simulink model "kinematic_obstacle_mpc"  (R2015b)
settings: Solver=FixedStepAuto  StartTime=0.0  StopTime=10.0  FixedStep=0.01  RelTol=1e-3
values from neighbouring files (symbols this model uses):
  goalX = 10    [KINEMATIC_MOTION_PLANNER.m]    (also in KINEMATIC_MOTION_PLANNER2.m = 15)
  goalY = 0    [KINEMATIC_MOTION_PLANNER.m]    (also in KINEMATIC_MOTION_PLANNER2.m)
  Lf = 1    [KINEMATIC_MOTION_PLANNER.m]    (also in KINEMATIC_MOTION_PLANNER2.m; KINEMATIC_STEP_MPC.m; KINEMATIC_VEHICLE_CONTROL.m; KINEMATIC_VEHICLE_SIM.m)
  Lr = 1    [KINEMATIC_MOTION_PLANNER.m]    (also in KINEMATIC_MOTION_PLANNER2.m; KINEMATIC_STEP_MPC.m; KINEMATIC_VEHICLE_CONTROL.m; KINEMATIC_VEHICLE_SIM.m)
  ObstacleX = 5    [KINEMATIC_MOTION_PLANNER.m]    (also in KINEMATIC_MOTION_PLANNER2.m = [5, 8,11])
  ObstacleY = 0    [KINEMATIC_MOTION_PLANNER.m]    (also in KINEMATIC_MOTION_PLANNER2.m = [0,-2.5,0])
  Psi0 = 0    [KINEMATIC_MOTION_PLANNER.m]    (also in KINEMATIC_MOTION_PLANNER2.m; KINEMATIC_STEP_MPC.m; KINEMATIC_VEHICLE_CONTROL.m; KINEMATIC_VEHICLE_SIM.m)
  V = 1    [KINEMATIC_MOTION_PLANNER.m]    (also in KINEMATIC_MOTION_PLANNER2.m; KINEMATIC_STEP_MPC.m; KINEMATIC_VEHICLE_CONTROL.m; KINEMATIC_VEHICLE_SIM.m = 5)
  X0 = 0    [KINEMATIC_MOTION_PLANNER.m]    (also in KINEMATIC_MOTION_PLANNER2.m; KINEMATIC_STEP_MPC.m; KINEMATIC_VEHICLE_CONTROL.m; KINEMATIC_VEHICLE_SIM.m)
  Y0 = 0    [KINEMATIC_MOTION_PLANNER.m]    (also in KINEMATIC_MOTION_PLANNER2.m; KINEMATIC_STEP_MPC.m; KINEMATIC_VEHICLE_CONTROL.m; KINEMATIC_VEHICLE_SIM.m)
settings Model: Creator=gebruiker  LastModifiedBy=gebruiker

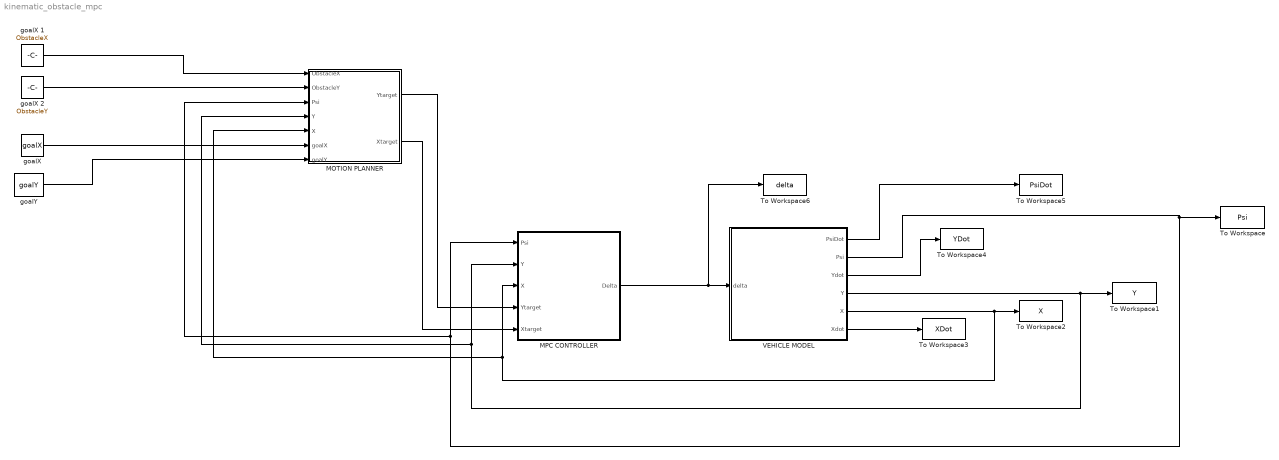
== system kinematic_obstacle_mpc ==
  MOTION PLANNER : Subsystem
  MPC CONTROLLER : Subsystem
  To Workspace : ToWorkspace  VariableName=Psi  SaveFormat=Structure With Time  SampleTime=-1
  To Workspace1 : ToWorkspace  VariableName=Y  SaveFormat=Structure With Time  SampleTime=-1
  To Workspace2 : ToWorkspace  VariableName=X  SaveFormat=Structure With Time  SampleTime=-1
  To Workspace3 : ToWorkspace  VariableName=XDot  SaveFormat=Structure With Time  SampleTime=-1
  To Workspace4 : ToWorkspace  VariableName=YDot  SaveFormat=Structure With Time  SampleTime=-1
  To Workspace5 : ToWorkspace  VariableName=PsiDot  SaveFormat=Structure With Time  SampleTime=-1
  To Workspace6 : ToWorkspace  VariableName=delta  SaveFormat=Structure With Time  SampleTime=-1
  VEHICLE MODEL : Subsystem
  "goalX " : Constant  Value=goalX
  goalX 1 : Constant  Value=ObstacleX
  goalX 2 : Constant  Value=ObstacleY
  "goalY " : Constant  Value=goalY
  wires:
  VEHICLE MODEL/1(PsiDot) -> To Workspace5/1
  VEHICLE MODEL/2(Psi) -> To Workspace/1, MOTION PLANNER/3("Psi "), MPC CONTROLLER/1(Psi)
  VEHICLE MODEL/3(Ydot) -> To Workspace4/1
  VEHICLE MODEL/4(Y) -> MOTION PLANNER/4("Y "), MPC CONTROLLER/2(Y), To Workspace1/1
  VEHICLE MODEL/6(Xdot) -> To Workspace3/1
  MPC CONTROLLER/1(Delta) -> To Workspace6/1, VEHICLE MODEL/1("delta ")
  VEHICLE MODEL/5(X) -> To Workspace2/1, MOTION PLANNER/5(X), MPC CONTROLLER/3(X)
  MOTION PLANNER/1(Ytarget) -> MPC CONTROLLER/4(Ytarget)
  MOTION PLANNER/2(Xtarget) -> MPC CONTROLLER/5(Xtarget)
  "goalX "/1 -> MOTION PLANNER/6(goalX)
  "goalY "/1 -> MOTION PLANNER/7("goalY ")
  goalX 2/1 -> MOTION PLANNER/2(ObstacleY)
  goalX 1/1 -> MOTION PLANNER/1(ObstacleX)

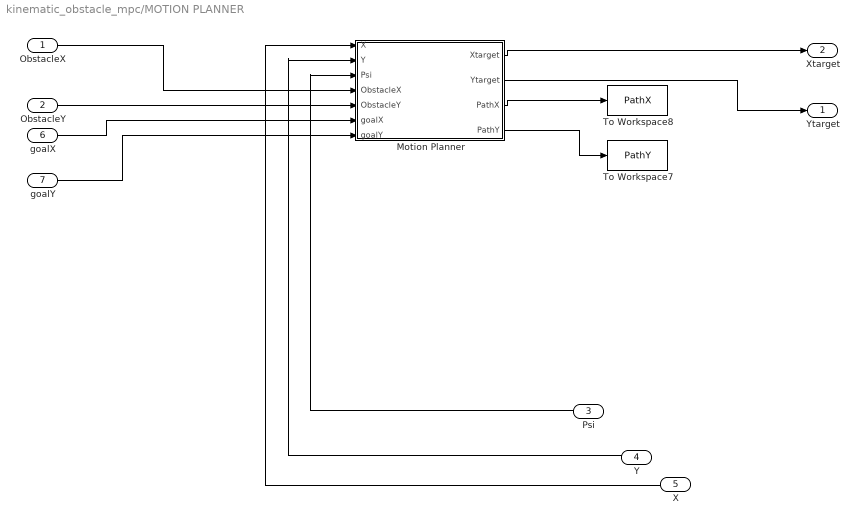
== system kinematic_obstacle_mpc/MOTION PLANNER ==
  ObstacleX : Inport
  ObstacleY : Inport  Port=2
  "Psi " : Inport  Port=3
  "Y " : Inport  Port=4
  X : Inport  Port=5
  goalX : Inport  Port=6
  "goalY " : Inport  Port=7
  Motion Planner : MATLAB Function  TreatAsAtomicUnit=on
  To Workspace7 : ToWorkspace  VariableName=PathY  SaveFormat=Structure With Time  SampleTime=-1
  To Workspace8 : ToWorkspace  VariableName=PathX  SaveFormat=Structure With Time  SampleTime=-1
  Ytarget : Outport
  Xtarget : Outport  Port=2
  wires:
  ObstacleY/1 -> Motion Planner/5(ObstacleY)
  Motion Planner/4(PathY) -> To Workspace7/1
  "Psi "/1 -> Motion Planner/3(Psi)
  "Y "/1 -> Motion Planner/2(Y)
  X/1 -> Motion Planner/1(X)
  Motion Planner/3(PathX) -> To Workspace8/1
  ObstacleX/1 -> Motion Planner/4(ObstacleX)
  Motion Planner/1(Xtarget) -> Xtarget/1
  Motion Planner/2(Ytarget) -> Ytarget/1
  goalX/1 -> Motion Planner/6(goalX)
  "goalY "/1 -> Motion Planner/7(goalY)

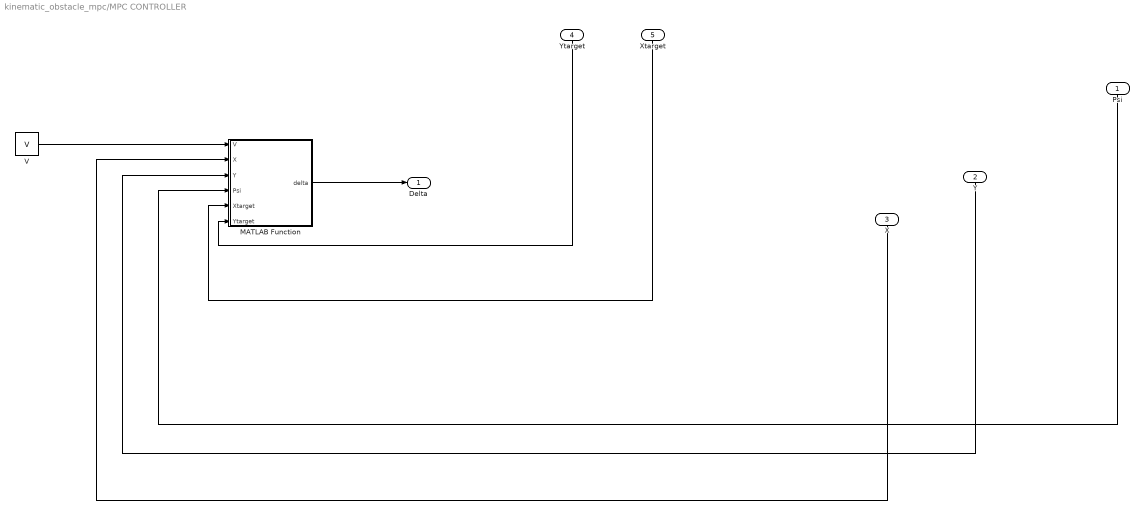
== system kinematic_obstacle_mpc/MPC CONTROLLER ==
  Psi : Inport
  Y : Inport  Port=2
  X : Inport  Port=3
  Ytarget : Inport  Port=4
  Xtarget : Inport  Port=5
  MATLAB Function : MATLAB Function  TreatAsAtomicUnit=on
  "V " : Constant  Value=V
  Delta : Outport
  wires:
  "V "/1 -> MATLAB Function/1(V)
  Y/1 -> MATLAB Function/3(Y)
  Psi/1 -> MATLAB Function/4(Psi)
  X/1 -> MATLAB Function/2(X)
  MATLAB Function/1(delta) -> Delta/1
  Xtarget/1 -> MATLAB Function/5(Xtarget)
  Ytarget/1 -> MATLAB Function/6(Ytarget)

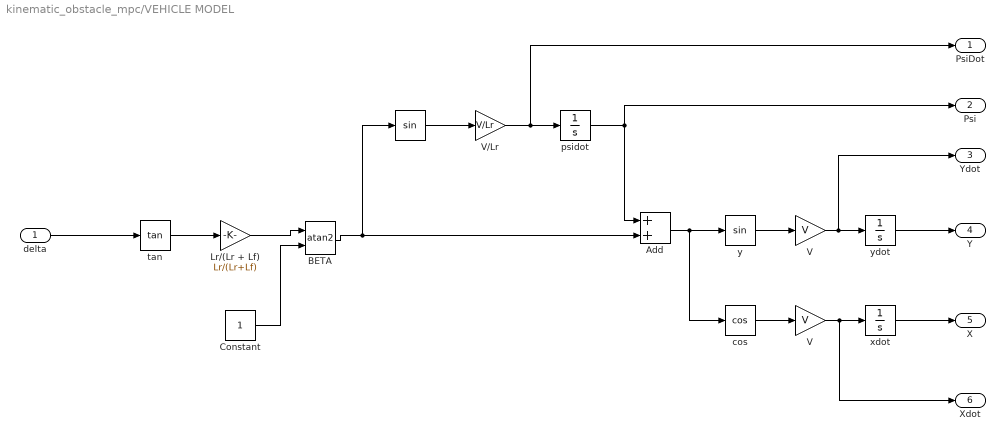
== system kinematic_obstacle_mpc/VEHICLE MODEL ==
  "delta " : Inport
  " " : Trigonometry
  Add : Sum
  BETA : Trigonometry  Operator=atan2
  Constant : Constant
  Lr/(Lr + Lf) : Gain  Gain=Lr/(Lr+Lf)
  V : Gain  Gain=V
  "V " : Gain  Gain=V
  V/Lr : Gain  Gain=V/Lr
  cos : Trigonometry  Operator=cos
  psidot : Integrator  InitialCondition=Psi0
  "tan " : Trigonometry  Operator=tan
  xdot : Integrator  InitialCondition=X0
  y : Trigonometry
  ydot : Integrator  InitialCondition=Y0
  PsiDot : Outport
  Psi : Outport  Port=2
  Ydot : Outport  Port=3
  Y : Outport  Port=4
  X : Outport  Port=5
  Xdot : Outport  Port=6
  wires:
  V/1 -> Ydot/1, ydot/1
  Lr/(Lr + Lf)/1 -> BETA/1
  BETA/1 -> Add/2, " "/1
  "V "/1 -> Xdot/1, xdot/1
  Add/1 -> cos/1, y/1
  xdot/1 -> X/1
  ydot/1 -> Y/1
  psidot/1 -> Psi/1, Add/1
  "delta "/1 -> "tan "/1
  V/Lr/1 -> PsiDot/1, psidot/1
  y/1 -> V/1
  " "/1 -> V/Lr/1
  "tan "/1 -> Lr/(Lr + Lf)/1
  cos/1 -> "V "/1
  Constant/1 -> BETA/2

== matlab function kinematic_obstacle_mpc/MOTION PLANNER/Motion Planner ==
  data: X input; Xtarget output; Y input; Psi input; ObstacleX input; ObstacleY input; Ytarget output; PathX output; PathY output; goalX input; goalY input
function [Xtarget, Ytarget, PathX,PathY] = Planner(X,Y,Psi,ObstacleX,ObstacleY,goalX,goalY)
%#codegen
R_Max = 3.5 % Max turning radius
obstcl_size = 2;

Robj = sqrt((ObstacleX-X)^2+(ObstacleY-Y)^2);
Rgoal = sqrt((goalX-X)^2+ (goalY-Y)^2);

if Robj < Rgoal
    if Robj < 2* R_Max
        theta = acos(Robj/(2*R_Max));
        thetas = linspace(-theta,theta, 21);
    else 
        thetas = linspace(0,2*pi,50)
    end
    
    dist_min = 1e9;
    theta_best = -100;
    x_opt = 0;
    y_opt = 0;
    for i = 1:length(thetas)
        thet = thetas(i);
        xt = Robj*cos(thet) + X;
        yt = Robj*sin(thet) + Y;
        distance = sqrt((goalX-xt)^2+(goalY-yt)^2);
        if (distance < dist_min) && (sqrt((ObstacleX-xt)^2+(ObstacleY-yt)^2) > obstcl_size)
            dist_min = distance;
            theta_best = thet;
            x_opt = xt;
            y_opt = yt;
        end   
    end
    Xtarget = x_opt;
    Ytarget = y_opt;
    PathX = [X,Xtarget,goalX];
    PathY = [Y,Ytarget,goalY];

else 
    Xtarget = goalX;
    Ytarget = goalY;
    PathX = [X,goalX,goalX];
    PathY = [Y,goalY,goalY];
end

end

== matlab function kinematic_obstacle_mpc/MPC CONTROLLER/MATLAB Function ==
  data: V input; delta output; X input; Y input; Psi input; Xtarget input; Ytarget input
function delta = fcn(V,X,Y,Psi,Xtarget,Ytarget)
%#codegen
% 
dt = 0.1;
R = [cos(Psi), -sin(Psi);sin(Psi),cos(Psi)];
Lmin = 1000;
delta_best = 0;
for delta = linspace(-pi/6,pi/6,21)
    dx = V*dt;
    dy = 2*V*delta*dt;
    drot = R*[dx;dy];
    Xfin = X + drot(1);
    Yfin = Y + drot(2);
    L = sqrt((Xtarget - Xfin)^2+(Ytarget - Yfin)^2);
    if L < Lmin
        Lmin = L;
        delta_best = delta;
    end
end
delta = delta_best;
end
